simulink model "torqueTest"  (R2020b)
settings: Solver=VariableStepAuto  StartTime=0.0  StopTime=4  FixedStep=0.5  RelTol=1e-3
values from neighbouring files (symbols this model uses):
  X = [x,y,z,Roll,Pitch,Yaw]    [T2RPY.m]
undefined symbols (not defined in the file or in its folder): Y, Z
libraries: sm_lib x75, nesl_utility x25
(part 2 of 2)

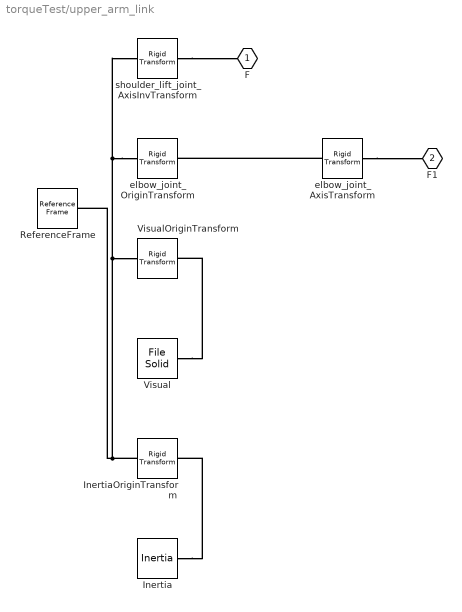
== system torqueTest/upper_arm_link ==
  Inertia : sm_lib/Body Elements/Inertia  InertiaType=Custom  Mass=12.877  MassUnits=kg  CenterOfMass=[0, 0, 0]  CenterOfMassUnits=m  MomentsOfInertia=[0.024695, 0.019038, 0.018496]  MomentsOfInertiaUnits=kg*m^2  ProductsOfInertia=[0.00066134, -6.8716e-08, -8.270400000000001e-09]  ProductsOfInertiaUnits=kg*m^2  GraphicType=None  MarkerShape=Inertia  MarkerSize=20  GraphicVisPropType=SimpleVisualProperties  GraphicDiffuseColor=[0.5 0.5 0.5]  GraphicSpecularColor=[0.5 0.5 0.5 1.0]  GraphicAmbientColor=[0.15 0.15 0.15 1.0]  GraphicEmissiveColor=[0.0 0.0 0.0 1.0]  GraphicShininess=75  GraphicOpacity=1.0
  InertiaOriginTransform : sm_lib/Frames and Transforms/Rigid Transform  TranslationMethod=Cartesian  TranslationStandardOffset=0  TranslationLengthUnit=m  TranslationStandardAxis=+Z  TranslationCartesianOffset=[-5.4357e-07, 0.0032767, 0.12625]  TranslationROffset=0  TranslationROffsetUnits=m  TranslationZOffset=0  TranslationZOffsetUnits=m  TranslationThetaOffset=0  TranslationThetaOffsetUnits=deg  RotationMethod=RotationSequence  RotationAngleUnits=deg  RotationStandardAxis=+Z  RotationAngle=0.0  RotationArbitraryAxis=[0 0 1]  FollAlignAxisA=+X  BaseAlignAxisA=+Y  FollAlignAxisB=+Y  BaseAlignAxisB=+Z  RotationSequenceAxes=BaseAxes  RotationSequence=XYZ  RotationSequenceAngles=[0, 0, 0]  RotationSequenceAnglesUnits=rad  RotationMatrix=[1 0 0; 0 1 0; 0 0 1]
  ReferenceFrame : sm_lib/Frames and Transforms/Reference Frame
  Visual : sm_lib/Body Elements/File Solid  ExtGeomFileName=ROCR6II_URDF_file/meshes/upper_arm_link.STL  UnitType=Custom  ExtGeomFileUnits=m  StepReaderType=HEX  ExportConvexHullGeometry=off  InertiaType=CalculateFromGeometry  Mass=0  MassUnits=kg  CenterOfMass=[0, 0, 0]  CenterOfMassUnits=m  MomentsOfInertia=[0, 0, 0]  MomentsOfInertiaUnits=kg*m^2  ProductsOfInertia=[0, 0, 0]  ProductsOfInertiaUnits=kg*m^2  BasedOnType=Density  Density=1000  DensityUnits=kg/m^3  DoExposeReferenceFrame=on  SerializedFrames=<Frames/>  GraphicType=FromGeometry  MarkerShape=Sphere  MarkerSize=10  GraphicVisPropType=SimpleVisualProperties  GraphicDiffuseColor=[0.7529400000000001, 0.7529400000000001, 0.7529400000000001]  GraphicSpecularColor=[0.5 0.5 0.5 1.0]  GraphicAmbientColor=[0.15 0.15 0.15 1.0]  GraphicEmissiveColor=[0.0 0.0 0.0 1.0]  GraphicShininess=75  GraphicOpacity=1
  VisualOriginTransform : sm_lib/Frames and Transforms/Rigid Transform  TranslationMethod=Cartesian  TranslationStandardOffset=0  TranslationLengthUnit=m  TranslationStandardAxis=+Z  TranslationCartesianOffset=[0, 0, 0]  TranslationROffset=0  TranslationROffsetUnits=m  TranslationZOffset=0  TranslationZOffsetUnits=m  TranslationThetaOffset=0  TranslationThetaOffsetUnits=deg  RotationMethod=RotationSequence  RotationAngleUnits=deg  RotationStandardAxis=+Z  RotationAngle=0.0  RotationArbitraryAxis=[0 0 1]  FollAlignAxisA=+X  BaseAlignAxisA=+Y  FollAlignAxisB=+Y  BaseAlignAxisB=+Z  RotationSequenceAxes=BaseAxes  RotationSequence=XYZ  RotationSequenceAngles=[0, 0, 0]  RotationSequenceAnglesUnits=rad  RotationMatrix=[1 0 0; 0 1 0; 0 0 1]
  elbow_joint_AxisTransform : sm_lib/Frames and Transforms/Rigid Transform  TranslationMethod=Cartesian  TranslationStandardOffset=0  TranslationLengthUnit=m  TranslationStandardAxis=+Z  TranslationCartesianOffset=[0, 0, 0]  TranslationROffset=0  TranslationROffsetUnits=m  TranslationZOffset=0  TranslationZOffsetUnits=m  TranslationThetaOffset=0  TranslationThetaOffsetUnits=deg  RotationMethod=ArbitraryAxis  RotationAngleUnits=rad  RotationStandardAxis=+Z  RotationAngle=1.570796326794897  RotationArbitraryAxis=[-1, 0, 0]  FollAlignAxisA=+X  BaseAlignAxisA=+Y  FollAlignAxisB=+Y  BaseAlignAxisB=+Z  RotationSequenceAxes=FollowerAxes  RotationSequence=XYX  RotationSequenceAngles=[0 0 0]  RotationSequenceAnglesUnits=deg  RotationMatrix=[1 0 0; 0 1 0; 0 0 1]
  elbow_joint_OriginTransform : sm_lib/Frames and Transforms/Rigid Transform  TranslationMethod=Cartesian  TranslationStandardOffset=0  TranslationLengthUnit=m  TranslationStandardAxis=+Z  TranslationCartesianOffset=[0, -0.102, 0.3]  TranslationROffset=0  TranslationROffsetUnits=m  TranslationZOffset=0  TranslationZOffsetUnits=m  TranslationThetaOffset=0  TranslationThetaOffsetUnits=deg  RotationMethod=RotationSequence  RotationAngleUnits=deg  RotationStandardAxis=+Z  RotationAngle=0.0  RotationArbitraryAxis=[0 0 1]  FollAlignAxisA=+X  BaseAlignAxisA=+Y  FollAlignAxisB=+Y  BaseAlignAxisB=+Z  RotationSequenceAxes=BaseAxes  RotationSequence=XYZ  RotationSequenceAngles=[0, 0, 0]  RotationSequenceAnglesUnits=rad  RotationMatrix=[1 0 0; 0 1 0; 0 0 1]
  shoulder_lift_joint_AxisInvTransform : sm_lib/Frames and Transforms/Rigid Transform  TranslationMethod=Cartesian  TranslationStandardOffset=0  TranslationLengthUnit=m  TranslationStandardAxis=+Z  TranslationCartesianOffset=[0, 0, 0]  TranslationROffset=0  TranslationROffsetUnits=m  TranslationZOffset=0  TranslationZOffsetUnits=m  TranslationThetaOffset=0  TranslationThetaOffsetUnits=deg  RotationMethod=ArbitraryAxis  RotationAngleUnits=rad  RotationStandardAxis=+Z  RotationAngle=1.570796326794897  RotationArbitraryAxis=[-1, 0, 0]  FollAlignAxisA=+X  BaseAlignAxisA=+Y  FollAlignAxisB=+Y  BaseAlignAxisB=+Z  RotationSequenceAxes=FollowerAxes  RotationSequence=XYX  RotationSequenceAngles=[0 0 0]  RotationSequenceAnglesUnits=deg  RotationMatrix=[1 0 0; 0 1 0; 0 0 1]
  F : PMIOPort  Side=Left
  F1 : PMIOPort  Port=2  Side=Right
  connections:
  Inertia/RConn1 -- InertiaOriginTransform/RConn1
  elbow_joint_OriginTransform/LConn1 -- shoulder_lift_joint_AxisInvTransform/LConn1 -- InertiaOriginTransform/LConn1 -- ReferenceFrame/RConn1 -- VisualOriginTransform/LConn1
  Visual/RConn1 -- VisualOriginTransform/RConn1
  elbow_joint_AxisTransform/RConn1 -- F1/RConn1
  elbow_joint_AxisTransform/LConn1 -- elbow_joint_OriginTransform/RConn1
  shoulder_lift_joint_AxisInvTransform/RConn1 -- F/RConn1

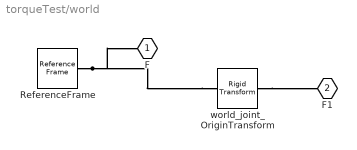
== system torqueTest/world ==
  ReferenceFrame : sm_lib/Frames and Transforms/Reference Frame
  world_joint_OriginTransform : sm_lib/Frames and Transforms/Rigid Transform  TranslationMethod=Cartesian  TranslationStandardOffset=0  TranslationLengthUnit=m  TranslationStandardAxis=+Z  TranslationCartesianOffset=[0, 0, 0]  TranslationROffset=0  TranslationROffsetUnits=m  TranslationZOffset=0  TranslationZOffsetUnits=m  TranslationThetaOffset=0  TranslationThetaOffsetUnits=deg  RotationMethod=RotationSequence  RotationAngleUnits=deg  RotationStandardAxis=+Z  RotationAngle=0.0  RotationArbitraryAxis=[0 0 1]  FollAlignAxisA=+X  BaseAlignAxisA=+Y  FollAlignAxisB=+Y  BaseAlignAxisB=+Z  RotationSequenceAxes=BaseAxes  RotationSequence=XYZ  RotationSequenceAngles=[3.1415926536, 3.1415926536, 0]  RotationSequenceAnglesUnits=rad  RotationMatrix=[1 0 0; 0 1 0; 0 0 1]
  F : PMIOPort  Side=Left
  F1 : PMIOPort  Port=2  Side=Right
  connections:
  world_joint_OriginTransform/LConn1 -- ReferenceFrame/RConn1 -- F/RConn1
  world_joint_OriginTransform/RConn1 -- F1/RConn1

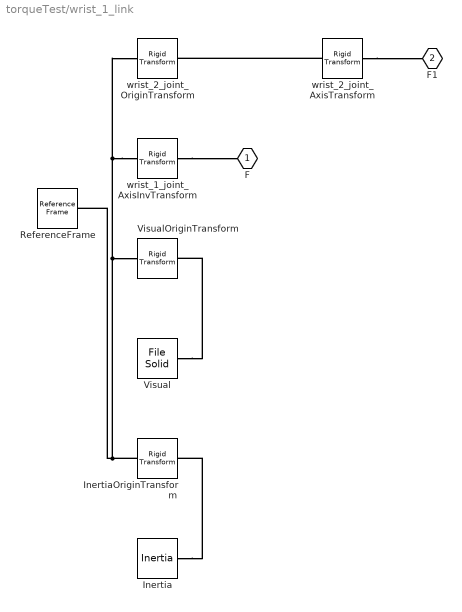
== system torqueTest/wrist_1_link ==
  Inertia : sm_lib/Body Elements/Inertia  InertiaType=Custom  Mass=3.1072  MassUnits=kg  CenterOfMass=[0, 0, 0]  CenterOfMassUnits=m  MomentsOfInertia=[0.0040287, 0.0039406, 0.0018825]  MomentsOfInertiaUnits=kg*m^2  ProductsOfInertia=[9.4145e-05, -2.3481e-09, -7.3158e-09]  ProductsOfInertiaUnits=kg*m^2  GraphicType=None  MarkerShape=Inertia  MarkerSize=20  GraphicVisPropType=SimpleVisualProperties  GraphicDiffuseColor=[0.5 0.5 0.5]  GraphicSpecularColor=[0.5 0.5 0.5 1.0]  GraphicAmbientColor=[0.15 0.15 0.15 1.0]  GraphicEmissiveColor=[0.0 0.0 0.0 1.0]  GraphicShininess=75  GraphicOpacity=1.0
  InertiaOriginTransform : sm_lib/Frames and Transforms/Rigid Transform  TranslationMethod=Cartesian  TranslationStandardOffset=0  TranslationLengthUnit=m  TranslationStandardAxis=+Z  TranslationCartesianOffset=[5.3079e-07, 0.087296, -0.010609]  TranslationROffset=0  TranslationROffsetUnits=m  TranslationZOffset=0  TranslationZOffsetUnits=m  TranslationThetaOffset=0  TranslationThetaOffsetUnits=deg  RotationMethod=RotationSequence  RotationAngleUnits=deg  RotationStandardAxis=+Z  RotationAngle=0.0  RotationArbitraryAxis=[0 0 1]  FollAlignAxisA=+X  BaseAlignAxisA=+Y  FollAlignAxisB=+Y  BaseAlignAxisB=+Z  RotationSequenceAxes=BaseAxes  RotationSequence=XYZ  RotationSequenceAngles=[0, 0, 0]  RotationSequenceAnglesUnits=rad  RotationMatrix=[1 0 0; 0 1 0; 0 0 1]
  ReferenceFrame : sm_lib/Frames and Transforms/Reference Frame
  Visual : sm_lib/Body Elements/File Solid  ExtGeomFileName=ROCR6II_URDF_file/meshes/wrist_1_link.STL  UnitType=Custom  ExtGeomFileUnits=m  StepReaderType=HEX  ExportConvexHullGeometry=off  InertiaType=CalculateFromGeometry  Mass=0  MassUnits=kg  CenterOfMass=[0, 0, 0]  CenterOfMassUnits=m  MomentsOfInertia=[0, 0, 0]  MomentsOfInertiaUnits=kg*m^2  ProductsOfInertia=[0, 0, 0]  ProductsOfInertiaUnits=kg*m^2  BasedOnType=Density  Density=1000  DensityUnits=kg/m^3  DoExposeReferenceFrame=on  SerializedFrames=<Frames/>  GraphicType=FromGeometry  MarkerShape=Sphere  MarkerSize=10  GraphicVisPropType=SimpleVisualProperties  GraphicDiffuseColor=[1, 1, 1]  GraphicSpecularColor=[0.5 0.5 0.5 1.0]  GraphicAmbientColor=[0.15 0.15 0.15 1.0]  GraphicEmissiveColor=[0.0 0.0 0.0 1.0]  GraphicShininess=75  GraphicOpacity=1
  VisualOriginTransform : sm_lib/Frames and Transforms/Rigid Transform  TranslationMethod=Cartesian  TranslationStandardOffset=0  TranslationLengthUnit=m  TranslationStandardAxis=+Z  TranslationCartesianOffset=[0, 0, 0]  TranslationROffset=0  TranslationROffsetUnits=m  TranslationZOffset=0  TranslationZOffsetUnits=m  TranslationThetaOffset=0  TranslationThetaOffsetUnits=deg  RotationMethod=RotationSequence  RotationAngleUnits=deg  RotationStandardAxis=+Z  RotationAngle=0.0  RotationArbitraryAxis=[0 0 1]  FollAlignAxisA=+X  BaseAlignAxisA=+Y  FollAlignAxisB=+Y  BaseAlignAxisB=+Z  RotationSequenceAxes=BaseAxes  RotationSequence=XYZ  RotationSequenceAngles=[0, 0, 0]  RotationSequenceAnglesUnits=rad  RotationMatrix=[1 0 0; 0 1 0; 0 0 1]
  wrist_1_joint_AxisInvTransform : sm_lib/Frames and Transforms/Rigid Transform  TranslationMethod=Cartesian  TranslationStandardOffset=0  TranslationLengthUnit=m  TranslationStandardAxis=+Z  TranslationCartesianOffset=[0, 0, 0]  TranslationROffset=0  TranslationROffsetUnits=m  TranslationZOffset=0  TranslationZOffsetUnits=m  TranslationThetaOffset=0  TranslationThetaOffsetUnits=deg  RotationMethod=ArbitraryAxis  RotationAngleUnits=rad  RotationStandardAxis=+Z  RotationAngle=1.570796326794897  RotationArbitraryAxis=[-1, 0, 0]  FollAlignAxisA=+X  BaseAlignAxisA=+Y  FollAlignAxisB=+Y  BaseAlignAxisB=+Z  RotationSequenceAxes=FollowerAxes  RotationSequence=XYX  RotationSequenceAngles=[0 0 0]  RotationSequenceAnglesUnits=deg  RotationMatrix=[1 0 0; 0 1 0; 0 0 1]
  wrist_2_joint_AxisTransform : sm_lib/Frames and Transforms/Rigid Transform  TranslationMethod=Cartesian  TranslationStandardOffset=0  TranslationLengthUnit=m  TranslationStandardAxis=+Z  TranslationCartesianOffset=[0, 0, 0]  TranslationROffset=0  TranslationROffsetUnits=m  TranslationZOffset=0  TranslationZOffsetUnits=m  TranslationThetaOffset=0  TranslationThetaOffsetUnits=deg  RotationMethod=ArbitraryAxis  RotationAngleUnits=rad  RotationStandardAxis=+Z  RotationAngle=0  RotationArbitraryAxis=[1, 0, 0]  FollAlignAxisA=+X  BaseAlignAxisA=+Y  FollAlignAxisB=+Y  BaseAlignAxisB=+Z  RotationSequenceAxes=FollowerAxes  RotationSequence=XYX  RotationSequenceAngles=[0 0 0]  RotationSequenceAnglesUnits=deg  RotationMatrix=[1 0 0; 0 1 0; 0 0 1]
  wrist_2_joint_OriginTransform : sm_lib/Frames and Transforms/Rigid Transform  TranslationMethod=Cartesian  TranslationStandardOffset=0  TranslationLengthUnit=m  TranslationStandardAxis=+Z  TranslationCartesianOffset=[0, 0.09, 0]  TranslationROffset=0  TranslationROffsetUnits=m  TranslationZOffset=0  TranslationZOffsetUnits=m  TranslationThetaOffset=0  TranslationThetaOffsetUnits=deg  RotationMethod=RotationSequence  RotationAngleUnits=deg  RotationStandardAxis=+Z  RotationAngle=0.0  RotationArbitraryAxis=[0 0 1]  FollAlignAxisA=+X  BaseAlignAxisA=+Y  FollAlignAxisB=+Y  BaseAlignAxisB=+Z  RotationSequenceAxes=BaseAxes  RotationSequence=XYZ  RotationSequenceAngles=[0, 0, 0]  RotationSequenceAnglesUnits=rad  RotationMatrix=[1 0 0; 0 1 0; 0 0 1]
  F : PMIOPort  Side=Left
  F1 : PMIOPort  Port=2  Side=Right
  connections:
  Inertia/RConn1 -- InertiaOriginTransform/RConn1
  wrist_1_joint_AxisInvTransform/LConn1 -- wrist_2_joint_OriginTransform/LConn1 -- InertiaOriginTransform/LConn1 -- ReferenceFrame/RConn1 -- VisualOriginTransform/LConn1
  Visual/RConn1 -- VisualOriginTransform/RConn1
  wrist_1_joint_AxisInvTransform/RConn1 -- F/RConn1
  wrist_2_joint_AxisTransform/RConn1 -- F1/RConn1
  wrist_2_joint_AxisTransform/LConn1 -- wrist_2_joint_OriginTransform/RConn1

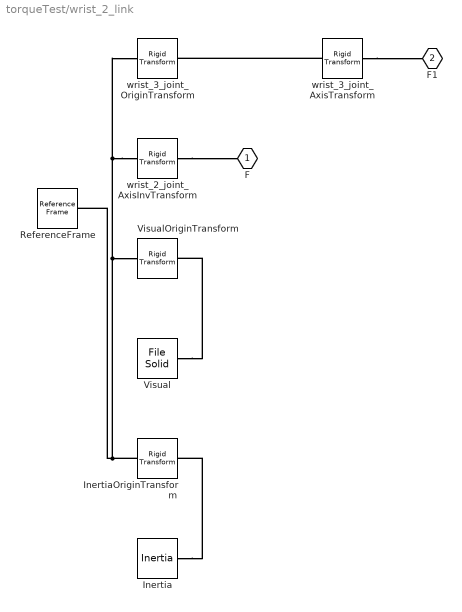
== system torqueTest/wrist_2_link ==
  Inertia : sm_lib/Body Elements/Inertia  InertiaType=Custom  Mass=3.1072  MassUnits=kg  CenterOfMass=[0, 0, 0]  CenterOfMassUnits=m  MomentsOfInertia=[0.0040287, 0.0018825, 0.0039406]  MomentsOfInertiaUnits=kg*m^2  ProductsOfInertia=[9.4145e-05, 7.3e-09, 2.3491e-09]  ProductsOfInertiaUnits=kg*m^2  GraphicType=None  MarkerShape=Inertia  MarkerSize=20  GraphicVisPropType=SimpleVisualProperties  GraphicDiffuseColor=[0.5 0.5 0.5]  GraphicSpecularColor=[0.5 0.5 0.5 1.0]  GraphicAmbientColor=[0.15 0.15 0.15 1.0]  GraphicEmissiveColor=[0.0 0.0 0.0 1.0]  GraphicShininess=75  GraphicOpacity=1.0
  InertiaOriginTransform : sm_lib/Frames and Transforms/Rigid Transform  TranslationMethod=Cartesian  TranslationStandardOffset=0  TranslationLengthUnit=m  TranslationStandardAxis=+Z  TranslationCartesianOffset=[-5.306000000000001e-07, -0.010609, 0.087296]  TranslationROffset=0  TranslationROffsetUnits=m  TranslationZOffset=0  TranslationZOffsetUnits=m  TranslationThetaOffset=0  TranslationThetaOffsetUnits=deg  RotationMethod=RotationSequence  RotationAngleUnits=deg  RotationStandardAxis=+Z  RotationAngle=0.0  RotationArbitraryAxis=[0 0 1]  FollAlignAxisA=+X  BaseAlignAxisA=+Y  FollAlignAxisB=+Y  BaseAlignAxisB=+Z  RotationSequenceAxes=BaseAxes  RotationSequence=XYZ  RotationSequenceAngles=[0, 0, 0]  RotationSequenceAnglesUnits=rad  RotationMatrix=[1 0 0; 0 1 0; 0 0 1]
  ReferenceFrame : sm_lib/Frames and Transforms/Reference Frame
  Visual : sm_lib/Body Elements/File Solid  ExtGeomFileName=ROCR6II_URDF_file/meshes/wrist_2_link.STL  UnitType=Custom  ExtGeomFileUnits=m  StepReaderType=HEX  ExportConvexHullGeometry=off  InertiaType=CalculateFromGeometry  Mass=0  MassUnits=kg  CenterOfMass=[0, 0, 0]  CenterOfMassUnits=m  MomentsOfInertia=[0, 0, 0]  MomentsOfInertiaUnits=kg*m^2  ProductsOfInertia=[0, 0, 0]  ProductsOfInertiaUnits=kg*m^2  BasedOnType=Density  Density=1000  DensityUnits=kg/m^3  DoExposeReferenceFrame=on  SerializedFrames=<Frames/>  GraphicType=FromGeometry  MarkerShape=Sphere  MarkerSize=10  GraphicVisPropType=SimpleVisualProperties  GraphicDiffuseColor=[1, 1, 1]  GraphicSpecularColor=[0.5 0.5 0.5 1.0]  GraphicAmbientColor=[0.15 0.15 0.15 1.0]  GraphicEmissiveColor=[0.0 0.0 0.0 1.0]  GraphicShininess=75  GraphicOpacity=1
  VisualOriginTransform : sm_lib/Frames and Transforms/Rigid Transform  TranslationMethod=Cartesian  TranslationStandardOffset=0  TranslationLengthUnit=m  TranslationStandardAxis=+Z  TranslationCartesianOffset=[0, 0, 0]  TranslationROffset=0  TranslationROffsetUnits=m  TranslationZOffset=0  TranslationZOffsetUnits=m  TranslationThetaOffset=0  TranslationThetaOffsetUnits=deg  RotationMethod=RotationSequence  RotationAngleUnits=deg  RotationStandardAxis=+Z  RotationAngle=0.0  RotationArbitraryAxis=[0 0 1]  FollAlignAxisA=+X  BaseAlignAxisA=+Y  FollAlignAxisB=+Y  BaseAlignAxisB=+Z  RotationSequenceAxes=BaseAxes  RotationSequence=XYZ  RotationSequenceAngles=[0, 0, 0]  RotationSequenceAnglesUnits=rad  RotationMatrix=[1 0 0; 0 1 0; 0 0 1]
  wrist_2_joint_AxisInvTransform : sm_lib/Frames and Transforms/Rigid Transform  TranslationMethod=Cartesian  TranslationStandardOffset=0  TranslationLengthUnit=m  TranslationStandardAxis=+Z  TranslationCartesianOffset=[0, 0, 0]  TranslationROffset=0  TranslationROffsetUnits=m  TranslationZOffset=0  TranslationZOffsetUnits=m  TranslationThetaOffset=0  TranslationThetaOffsetUnits=deg  RotationMethod=ArbitraryAxis  RotationAngleUnits=rad  RotationStandardAxis=+Z  RotationAngle=0  RotationArbitraryAxis=[1, 0, 0]  FollAlignAxisA=+X  BaseAlignAxisA=+Y  FollAlignAxisB=+Y  BaseAlignAxisB=+Z  RotationSequenceAxes=FollowerAxes  RotationSequence=XYX  RotationSequenceAngles=[0 0 0]  RotationSequenceAnglesUnits=deg  RotationMatrix=[1 0 0; 0 1 0; 0 0 1]
  wrist_3_joint_AxisTransform : sm_lib/Frames and Transforms/Rigid Transform  TranslationMethod=Cartesian  TranslationStandardOffset=0  TranslationLengthUnit=m  TranslationStandardAxis=+Z  TranslationCartesianOffset=[0, 0, 0]  TranslationROffset=0  TranslationROffsetUnits=m  TranslationZOffset=0  TranslationZOffsetUnits=m  TranslationThetaOffset=0  TranslationThetaOffsetUnits=deg  RotationMethod=ArbitraryAxis  RotationAngleUnits=rad  RotationStandardAxis=+Z  RotationAngle=1.570796326794897  RotationArbitraryAxis=[-1, 0, 0]  FollAlignAxisA=+X  BaseAlignAxisA=+Y  FollAlignAxisB=+Y  BaseAlignAxisB=+Z  RotationSequenceAxes=FollowerAxes  RotationSequence=XYX  RotationSequenceAngles=[0 0 0]  RotationSequenceAnglesUnits=deg  RotationMatrix=[1 0 0; 0 1 0; 0 0 1]
  wrist_3_joint_OriginTransform : sm_lib/Frames and Transforms/Rigid Transform  TranslationMethod=Cartesian  TranslationStandardOffset=0  TranslationLengthUnit=m  TranslationStandardAxis=+Z  TranslationCartesianOffset=[0, 0, 0.09]  TranslationROffset=0  TranslationROffsetUnits=m  TranslationZOffset=0  TranslationZOffsetUnits=m  TranslationThetaOffset=0  TranslationThetaOffsetUnits=deg  RotationMethod=RotationSequence  RotationAngleUnits=deg  RotationStandardAxis=+Z  RotationAngle=0.0  RotationArbitraryAxis=[0 0 1]  FollAlignAxisA=+X  BaseAlignAxisA=+Y  FollAlignAxisB=+Y  BaseAlignAxisB=+Z  RotationSequenceAxes=BaseAxes  RotationSequence=XYZ  RotationSequenceAngles=[0, 0, 0]  RotationSequenceAnglesUnits=rad  RotationMatrix=[1 0 0; 0 1 0; 0 0 1]
  F : PMIOPort  Side=Left
  F1 : PMIOPort  Port=2  Side=Right
  connections:
  Inertia/RConn1 -- InertiaOriginTransform/RConn1
  wrist_2_joint_AxisInvTransform/LConn1 -- wrist_3_joint_OriginTransform/LConn1 -- InertiaOriginTransform/LConn1 -- ReferenceFrame/RConn1 -- VisualOriginTransform/LConn1
  Visual/RConn1 -- VisualOriginTransform/RConn1
  wrist_2_joint_AxisInvTransform/RConn1 -- F/RConn1
  wrist_3_joint_AxisTransform/RConn1 -- F1/RConn1
  wrist_3_joint_AxisTransform/LConn1 -- wrist_3_joint_OriginTransform/RConn1

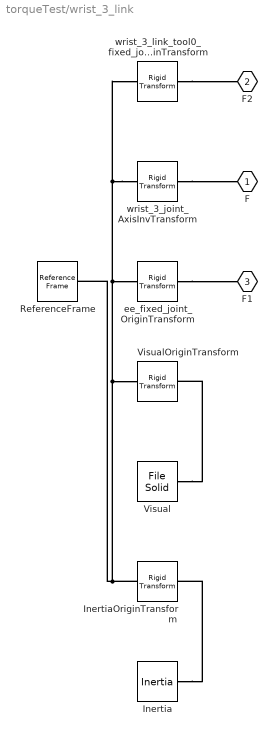
== system torqueTest/wrist_3_link ==
  Inertia : sm_lib/Body Elements/Inertia  InertiaType=Custom  Mass=0.59141  MassUnits=kg  CenterOfMass=[0, 0, 0]  CenterOfMassUnits=m  MomentsOfInertia=[0.0002476, 0.00040058, 0.00024889]  MomentsOfInertiaUnits=kg*m^2  ProductsOfInertia=[4.9238e-06, 1.3425e-10, -2.2015e-14]  ProductsOfInertiaUnits=kg*m^2  GraphicType=None  MarkerShape=Inertia  MarkerSize=20  GraphicVisPropType=SimpleVisualProperties  GraphicDiffuseColor=[0.5 0.5 0.5]  GraphicSpecularColor=[0.5 0.5 0.5 1.0]  GraphicAmbientColor=[0.15 0.15 0.15 1.0]  GraphicEmissiveColor=[0.0 0.0 0.0 1.0]  GraphicShininess=75  GraphicOpacity=1.0
  InertiaOriginTransform : sm_lib/Frames and Transforms/Rigid Transform  TranslationMethod=Cartesian  TranslationStandardOffset=0  TranslationLengthUnit=m  TranslationStandardAxis=+Z  TranslationCartesianOffset=[-1.7174e-09, 0.064961, 2.5473e-05]  TranslationROffset=0  TranslationROffsetUnits=m  TranslationZOffset=0  TranslationZOffsetUnits=m  TranslationThetaOffset=0  TranslationThetaOffsetUnits=deg  RotationMethod=RotationSequence  RotationAngleUnits=deg  RotationStandardAxis=+Z  RotationAngle=0.0  RotationArbitraryAxis=[0 0 1]  FollAlignAxisA=+X  BaseAlignAxisA=+Y  FollAlignAxisB=+Y  BaseAlignAxisB=+Z  RotationSequenceAxes=BaseAxes  RotationSequence=XYZ  RotationSequenceAngles=[0, 0, 0]  RotationSequenceAnglesUnits=rad  RotationMatrix=[1 0 0; 0 1 0; 0 0 1]
  ReferenceFrame : sm_lib/Frames and Transforms/Reference Frame
  Visual : sm_lib/Body Elements/File Solid  ExtGeomFileName=ROCR6II_URDF_file/meshes/wrist_3_link.STL  UnitType=Custom  ExtGeomFileUnits=m  StepReaderType=HEX  ExportConvexHullGeometry=off  InertiaType=CalculateFromGeometry  Mass=0  MassUnits=kg  CenterOfMass=[0, 0, 0]  CenterOfMassUnits=m  MomentsOfInertia=[0, 0, 0]  MomentsOfInertiaUnits=kg*m^2  ProductsOfInertia=[0, 0, 0]  ProductsOfInertiaUnits=kg*m^2  BasedOnType=Density  Density=1000  DensityUnits=kg/m^3  DoExposeReferenceFrame=on  SerializedFrames=<Frames/>  GraphicType=FromGeometry  MarkerShape=Sphere  MarkerSize=10  GraphicVisPropType=SimpleVisualProperties  GraphicDiffuseColor=[0.7529400000000001, 0.7529400000000001, 0.7529400000000001]  GraphicSpecularColor=[0.5 0.5 0.5 1.0]  GraphicAmbientColor=[0.15 0.15 0.15 1.0]  GraphicEmissiveColor=[0.0 0.0 0.0 1.0]  GraphicShininess=75  GraphicOpacity=1
  VisualOriginTransform : sm_lib/Frames and Transforms/Rigid Transform  TranslationMethod=Cartesian  TranslationStandardOffset=0  TranslationLengthUnit=m  TranslationStandardAxis=+Z  TranslationCartesianOffset=[0, 0, 0]  TranslationROffset=0  TranslationROffsetUnits=m  TranslationZOffset=0  TranslationZOffsetUnits=m  TranslationThetaOffset=0  TranslationThetaOffsetUnits=deg  RotationMethod=RotationSequence  RotationAngleUnits=deg  RotationStandardAxis=+Z  RotationAngle=0.0  RotationArbitraryAxis=[0 0 1]  FollAlignAxisA=+X  BaseAlignAxisA=+Y  FollAlignAxisB=+Y  BaseAlignAxisB=+Z  RotationSequenceAxes=BaseAxes  RotationSequence=XYZ  RotationSequenceAngles=[0, 0, 0]  RotationSequenceAnglesUnits=rad  RotationMatrix=[1 0 0; 0 1 0; 0 0 1]
  ee_fixed_joint_OriginTransform : sm_lib/Frames and Transforms/Rigid Transform  TranslationMethod=Cartesian  TranslationStandardOffset=0  TranslationLengthUnit=m  TranslationStandardAxis=+Z  TranslationCartesianOffset=[0, 0.09, 0]  TranslationROffset=0  TranslationROffsetUnits=m  TranslationZOffset=0  TranslationZOffsetUnits=m  TranslationThetaOffset=0  TranslationThetaOffsetUnits=deg  RotationMethod=RotationSequence  RotationAngleUnits=deg  RotationStandardAxis=+Z  RotationAngle=0.0  RotationArbitraryAxis=[0 0 1]  FollAlignAxisA=+X  BaseAlignAxisA=+Y  FollAlignAxisB=+Y  BaseAlignAxisB=+Z  RotationSequenceAxes=BaseAxes  RotationSequence=XYZ  RotationSequenceAngles=[0, 0, 1.57079632679]  RotationSequenceAnglesUnits=rad  RotationMatrix=[1 0 0; 0 1 0; 0 0 1]
  wrist_3_joint_AxisInvTransform : sm_lib/Frames and Transforms/Rigid Transform  TranslationMethod=Cartesian  TranslationStandardOffset=0  TranslationLengthUnit=m  TranslationStandardAxis=+Z  TranslationCartesianOffset=[0, 0, 0]  TranslationROffset=0  TranslationROffsetUnits=m  TranslationZOffset=0  TranslationZOffsetUnits=m  TranslationThetaOffset=0  TranslationThetaOffsetUnits=deg  RotationMethod=ArbitraryAxis  RotationAngleUnits=rad  RotationStandardAxis=+Z  RotationAngle=1.570796326794897  RotationArbitraryAxis=[-1, 0, 0]  FollAlignAxisA=+X  BaseAlignAxisA=+Y  FollAlignAxisB=+Y  BaseAlignAxisB=+Z  RotationSequenceAxes=FollowerAxes  RotationSequence=XYX  RotationSequenceAngles=[0 0 0]  RotationSequenceAnglesUnits=deg  RotationMatrix=[1 0 0; 0 1 0; 0 0 1]
  wrist_3_link_tool0_fixed_joint_OriginTransform : sm_lib/Frames and Transforms/Rigid Transform  TranslationMethod=Cartesian  TranslationStandardOffset=0  TranslationLengthUnit=m  TranslationStandardAxis=+Z  TranslationCartesianOffset=[0, 0.082, 0]  TranslationROffset=0  TranslationROffsetUnits=m  TranslationZOffset=0  TranslationZOffsetUnits=m  TranslationThetaOffset=0  TranslationThetaOffsetUnits=deg  RotationMethod=RotationSequence  RotationAngleUnits=deg  RotationStandardAxis=+Z  RotationAngle=0.0  RotationArbitraryAxis=[0 0 1]  FollAlignAxisA=+X  BaseAlignAxisA=+Y  FollAlignAxisB=+Y  BaseAlignAxisB=+Z  RotationSequenceAxes=BaseAxes  RotationSequence=XYZ  RotationSequenceAngles=[-1.57079632679, 0, 0]  RotationSequenceAnglesUnits=rad  RotationMatrix=[1 0 0; 0 1 0; 0 0 1]
  F : PMIOPort  Side=Left
  F2 : PMIOPort  Port=2  Side=Right
  F1 : PMIOPort  Port=3  Side=Right
  connections:
  Inertia/RConn1 -- InertiaOriginTransform/RConn1
  wrist_3_joint_AxisInvTransform/LConn1 -- wrist_3_link_tool0_fixed_joint_OriginTransform/LConn1 -- InertiaOriginTransform/LConn1 -- ReferenceFrame/RConn1 -- VisualOriginTransform/LConn1 -- ee_fixed_joint_OriginTransform/LConn1
  Visual/RConn1 -- VisualOriginTransform/RConn1
  ee_fixed_joint_OriginTransform/RConn1 -- F1/RConn1
  wrist_3_joint_AxisInvTransform/RConn1 -- F/RConn1
  wrist_3_link_tool0_fixed_joint_OriginTransform/RConn1 -- F2/RConn1

== matlab function torqueTest/Subsystem/trToRPY1 ==
  data: T input; X output
function  X=Tr2Pos(T)
%#codegen
coder.extrinsic('disp'); %Declare disp as extrinsic
    %% 求末端位置
    x=T(1,4);y=T(2,4);z=T(3,4);
    %% 根据X-Y-Z固定角计算
    R=T;rpy=[0,0,0];
    if abs(abs(R(3,1)) - 1) < 0.000001  % when |R31| == 1
    % singularity
        rpy(1) = 0;     % roll is zero
        if R(3,1) < 0
            rpy(3) = -atan2(R(1,2), R(1,3));  % R-Y
        else
            rpy(3) = atan2(-R(1,2), -R(1,3));  % R+Y
        end
        rpy(2) = -asin(R(3,1));
    else
        rpy(1) = atan2(R(3,2), R(3,3));  % R
        rpy(3) = atan2(R(2,1), R(1,1));  % Y

        [~,k] = max(abs( [R(1,1) R(2,1) R(3,2) R(3,3)] ));
        switch k
            case 1
                rpy(2) = -atan(R(3,1)*cos(rpy(3))/R(1,1));
            case 2
                rpy(2) = -atan(R(3,1)*sin(rpy(3))/R(2,1));
            case 3
                rpy(2) = -atan(R(3,1)*sin(rpy(1))/R(3,2));
            case 4
                rpy(2) = -atan(R(3,1)*cos(rpy(1))/R(3,3));
        end
    end
%     RPY=rpy*180/pi;
    RPY=rpy;
    Roll=RPY(1);Pitch=RPY(2);Yaw=RPY(3);
    X=[x,y,z,Roll,Pitch,Yaw];
end

== matlab function torqueTest/Subsystem1/J_0 ==
  data: q input; J output
function J = J(q)
q1=q(1);q2=q(2);q3=q(3);q4=q(4);q5=q(5);q6=q(6);
%J
%    J = J(Q1,Q2,Q3,Q4,Q5)

%    This function was generated by the Symbolic Math Toolbox version 8.6.
%    07-Dec-2021 11:30:25

t2 = cos(q1);
t3 = cos(q2);
t4 = cos(q3);
t5 = cos(q4);
t6 = cos(q5);
t7 = sin(q1);
t8 = sin(q2);
t9 = sin(q3);
t10 = sin(q4);
t11 = sin(q5);
t12 = q2+q3+q4;
t13 = cos(t12);
t14 = sin(t12);
t15 = -t2;
t16 = t6.*(3.9e+1./4.0e+2);
t17 = t5.*(5.7e+1./5.0e+2);
t18 = t10.*(5.7e+1./5.0e+2);
t20 = t5.*t11.*(3.9e+1./4.0e+2);
t21 = t10.*t11.*(3.9e+1./4.0e+2);
t19 = -t18;
t22 = -t20;
t23 = t16+1.065e-1;
t24 = t17+t21;
t25 = t18+t22;
t26 = t4.*t24;
t27 = t9.*t24;
t32 = t19+t20+2.37e+2./1.0e+3;
t28 = t4.*t25;
t29 = t9.*t25;
t30 = -t27;
t33 = t4.*t32;
t34 = t9.*t32;
t31 = -t29;
t35 = t27+t28;
t40 = t26+t34;
t41 = t30+t33;
t44 = -t8.*(t27-t33);
t36 = t26+t31;
t37 = t8.*t35;
t42 = t3.*t40;
t43 = t8.*t40;
t46 = t41+3.3e+1./1.25e+2;
t38 = t3.*t36;
t39 = -t37;
t45 = -t43;
t47 = t3.*t46;
t48 = t8.*t46;
t50 = t42+t44;
t49 = t38+t39;
t51 = t42+t48;
t52 = t45+t47;
J = reshape([t2.*t23-t7.*(t43-t47),t7.*t23+t2.*(t43-t47),0.0,0.0,0.0,1.0,t2.*t51,t7.*t51,t43-t47,t7,t15,0.0,t2.*t50,t7.*t50,t43+t3.*(t27-t33),t7,t15,0.0,-t2.*(t37-t38),-t7.*(t37-t38),t3.*t35+t8.*t36,t7,t15,0.0,t7.*t11.*(-3.9e+1./4.0e+2)-t2.*t6.*t13.*(3.9e+1./4.0e+2),t2.*t11.*(3.9e+1./4.0e+2)-t6.*t7.*t13.*(3.9e+1./4.0e+2),t6.*t14.*(-3.9e+1./4.0e+2),t2.*t14,t7.*t14,-t13,0.0,0.0,0.0,t6.*t7+t11.*t13.*t15,t6.*t15-t7.*t11.*t13,-t11.*t14],[6,6]);


end

== matlab function torqueTest/Subsystem1/J_1 ==
  data: phi input; JaDown3 output; theta input; xi input; J input
function JaDown3 = Jana(phi,theta,xi,J)
om2eulmat=[cos(theta)*cos(xi), -sin(xi), 0;
    cos(theta)*sin(xi),  cos(xi), 0;
    -sin(theta),       0, 1];
omega=J(4:6,:);
JaDown3 = om2eulmat\omega;
end

== matlab function torqueTest/Subsystem1/MATLAB Function ==
  data: JaDown3 input; Jana output; J input
function Jana = fcn(JaDown3,J)
Jana=[J(1:3,:);JaDown3];
end

== matlab function torqueTest/Subsystem1/MATLAB Function1 ==
  data: Jana input; Jadot input; Janadot output; Janaold input
function Janadot = fcn(Jana,Jadot,Janaold)
Jadown3 = Jana - Janaold;
Janadot=[Jadot(1:3,:);Jadown3(4:6,:)];
end

== matlab function torqueTest/Subsystem1/MATLAB Function2 ==
  data: Jana input; Janadot input; dq input; ddX output; ddq input
function ddX = getddX(Jana,Janadot,dq,ddq)
ddX = Janadot * dq + Jana * ddq;

== matlab function torqueTest/Subsystem1/MATLAB Function3 ==
  data: Jana input; dX output; dq input
function dX = getdX(Jana,dq)
dX=Jana*dq;

== matlab function torqueTest/Subsystem1/Pdot1 ==
  data: q input; qdot input; Jadot output
function Jadot = Jadot(q,qdot)
%JADOT
%    JADOT = JADOT(Q1,Q2,Q3,Q4,Q5,Q1DOT,Q2DOT,Q3DOT,Q4DOT,Q5DOT)

%    This function was generated by the Symbolic Math Toolbox version 8.6.
%    07-Dec-2021 14:58:16
q1=q(1);q2=q(2);q3=q(3);q4=q(4);q5=q(5);q6=q(6);
q1dot=qdot(1);q2dot=qdot(2);q3dot=qdot(3);q4dot=qdot(4);q5dot=qdot(5);q6dot=qdot(6);
t2 = cos(q1);
t3 = cos(q2);
t4 = cos(q3);
t5 = cos(q4);
t6 = cos(q5);
t7 = sin(q1);
t8 = sin(q2);
t9 = sin(q3);
t10 = sin(q4);
t11 = sin(q5);
t12 = q2+q3+q4;
t13 = q2dot+q3dot+q4dot;
t14 = cos(t12);
t15 = sin(t12);
t16 = t6.*(3.9e+1./4.0e+2);
t17 = t5.*(5.7e+1./5.0e+2);
t18 = t10.*(5.7e+1./5.0e+2);
t22 = t5.*t11.*(3.9e+1./4.0e+2);
t23 = t10.*t11.*(3.9e+1./4.0e+2);
t24 = q4dot.*t10.*(-5.7e+1./5.0e+2);
t30 = q5dot.*t5.*t6.*(-3.9e+1./4.0e+2);
t19 = -t18;
t20 = q4dot.*t17;
t21 = q4dot.*t18;
t25 = -t22;
t26 = q5dot.*t5.*t16;
t27 = q4dot.*t22;
t28 = q5dot.*t10.*t16;
t29 = q4dot.*t23;
t31 = t16+1.065e-1;
t32 = t17+t23;
t33 = t18+t25;
t34 = t4.*t32;
t35 = t9.*t32;
t46 = t19+t22+2.37e+2./1.0e+3;
t51 = t20+t29+t30;
t52 = t24+t27+t28;
t36 = q3dot.*t34;
t37 = q3dot.*t35;
t38 = t4.*t33;
t39 = t9.*t33;
t42 = -t35;
t47 = t4.*t46;
t48 = t9.*t46;
t53 = t4.*t51;
t54 = t4.*t52;
t55 = t9.*t51;
t56 = t9.*t52;
t40 = q3dot.*t38;
t41 = q3dot.*t39;
t43 = -t37;
t44 = -t39;
t49 = q3dot.*t47;
t50 = q3dot.*t48;
t57 = -t54;
t58 = -t55;
t59 = t35+t38;
t66 = t34+t48;
t67 = t42+t47;
t72 = -t8.*(t35-t47);
t75 = -q2dot.*t3.*(t35-t47);
t45 = -t41;
t60 = t34+t44;
t61 = t8.*t59;
t62 = q2dot.*t3.*t59;
t68 = t3.*t66;
t69 = t8.*t66;
t76 = t67+3.3e+1./1.25e+2;
t85 = t37+t40+t55+t57;
t89 = t36+t50+t53+t56;
t92 = t43+t49+t54+t58;
t94 = -t3.*(t37-t49+t55+t57);
t95 = -t8.*(t37-t49+t55+t57);
t63 = t3.*t60;
t64 = -t61;
t65 = q2dot.*t8.*t60;
t70 = q2dot.*t69;
t71 = q2dot.*t68;
t73 = -t69;
t77 = t3.*t76;
t78 = t8.*t76;
t82 = t68+t72;
t84 = t36+t45+t53+t56;
t87 = t3.*t85;
t90 = t3.*t89;
t91 = t8.*t89;
t74 = -t70;
t79 = q2dot.*t78;
t80 = q2dot.*t77;
t81 = t63+t64;
t83 = t68+t78;
t86 = t73+t77;
t88 = t8.*t84;
t93 = -t91;
t96 = t62+t65+t87+t88;
t97 = t74+t75+t93+t94;
t98 = t71+t79+t90+t95;
t99 = t74+t80+t93+t94;
Jadot = reshape([-t7.*t98-q5dot.*t2.*t11.*(3.9e+1./4.0e+2)-q1dot.*t7.*t31-q1dot.*t2.*(t69-t77),t2.*t98-q5dot.*t7.*t11.*(3.9e+1./4.0e+2)+q1dot.*t2.*t31-q1dot.*t7.*(t69-t77),0.0,-t2.*(t70-t80+t91+t3.*(t37-t49+t55+t57))-q1dot.*t7.*t83,-t7.*(t70-t80+t91+t3.*(t37-t49+t55+t57))+q1dot.*t2.*t83,t98,-t2.*(t70+t91+t3.*(t37-t49+t55+t57)+q2dot.*t3.*(t35-t47))-q1dot.*t7.*t82,-t7.*(t70+t91+t3.*(t37-t49+t55+t57)+q2dot.*t3.*(t35-t47))+q1dot.*t2.*t82,t71+t90+t95+q2dot.*t72,-t2.*t96+q1dot.*t7.*(t61-t63),-t7.*t96-q1dot.*t2.*(t61-t63),q2dot.*t63+q2dot.*t64+t3.*t84-t8.*t85,q1dot.*t2.*t11.*(-3.9e+1./4.0e+2)-q5dot.*t6.*t7.*(3.9e+1./4.0e+2)+q5dot.*t2.*t11.*t14.*(3.9e+1./4.0e+2)+q1dot.*t7.*t14.*t16+t2.*t13.*t15.*t16,q1dot.*t7.*t11.*(-3.9e+1./4.0e+2)+q5dot.*t2.*t16-q1dot.*t2.*t6.*t14.*(3.9e+1./4.0e+2)+q5dot.*t7.*t11.*t14.*(3.9e+1./4.0e+2)+t7.*t13.*t15.*t16,q5dot.*t11.*t15.*(3.9e+1./4.0e+2)-t6.*t13.*t14.*(3.9e+1./4.0e+2),0.0,0.0,0.0],[3,6]);

end

== matlab function torqueTest/Subsystem1/T ==
  data: q input; T output
function T = transion(q)
q1=q(1);q2=q(2);q3=q(3);q4=q(4);q5=q(5);q6=q(6);
t2 = cos(q1);
t3 = cos(q2);
t4 = cos(q3);
t5 = cos(q4);
t6 = cos(q5);
t7 = cos(q6);
t8 = sin(q1);
t9 = sin(q2);
t10 = sin(q3);
t11 = sin(q4);
t12 = sin(q5);
t13 = sin(q6);
t14 = t2.*t3;
t15 = t3.*t4;
t16 = t2.*t6;
t17 = t2.*t9;
t18 = t3.*t8;
t19 = t3.*t10;
t20 = t4.*t9;
t21 = t2.*t12;
t22 = t6.*t8;
t23 = t8.*t9;
t24 = t9.*t10;
t25 = t8.*t12;
t42 = t2.*6.123233995736766e-17;
t43 = t6.*6.123233995736766e-17;
t44 = t8.*6.123233995736766e-17;
t45 = t12.*6.123233995736766e-17;
t26 = -t23;
t27 = -t24;
t28 = -t25;
t29 = t19+t20;
t46 = -t42;
t47 = t14.*6.123233995736766e-17;
t48 = t17.*6.123233995736766e-17;
t49 = t18.*6.123233995736766e-17;
t50 = t23.*6.123233995736766e-17;
t30 = t15+t27;
t31 = t5.*t29;
t32 = t11.*t29;
t51 = -t50;
t52 = t17+t49;
t53 = t18+t48;
t55 = t26+t47;
t33 = t5.*t30;
t34 = t11.*t30;
t35 = -t32;
t54 = t14+t51;
t56 = t10.*t52;
t57 = t10.*t53;
t58 = t4.*t52;
t59 = t4.*t53;
t62 = t10.*t55;
t63 = t4.*t55;
t36 = -t33;
t37 = t31+t34;
t38 = t33+t35;
t60 = t10.*t54;
t61 = t4.*t54;
t65 = -t63;
t70 = t59+t62;
t39 = t6.*t37;
t40 = t12.*t37;
t64 = -t61;
t66 = t6.*(t32+t36).*(-6.123233995736766e-17);
t67 = t12.*(t32+t36).*(-6.123233995736766e-17);
t68 = t58+t60;
t69 = t32+t36+3.749399456654644e-33;
t72 = t57+t65;
t75 = t5.*t70;
t76 = t11.*t70;
t41 = -t40;
t71 = t56+t64;
t73 = t5.*t68;
t74 = t11.*t68;
t79 = t5.*t72;
t80 = t11.*t72;
t83 = t39+t45+t67;
t77 = t5.*t71;
t78 = t11.*t71;
t82 = -t80;
t84 = t41+t43+t66;
t87 = t76+t79;
t81 = -t78;
t85 = t74+t77;
t90 = t75+t82;
t96 = t12.*t87.*6.123233995736766e-17;
t98 = t6.*t87.*6.123233995736766e-17;
t99 = t46+t87;
t86 = t73+t81;
t88 = t6.*t85;
t89 = t12.*t85;
t91 = t6.*t90;
t92 = t12.*t90;
t93 = -t91;
t94 = t44+t86;
t95 = t45.*t86;
t97 = t43.*t86;
t100 = t6.*t86.*(-6.123233995736766e-17);
t103 = t16+t92+t98;
t101 = t22+t89+t100;
t102 = t28+t88+t95;
t104 = t21+t93+t96;
T = reshape([-t13.*t94+t13.*(t22+t89-t97).*6.123233995736766e-17-t7.*(-t25+t88+t12.*t86.*6.123233995736766e-17),t13.*t103.*(-6.123233995736766e-17)-t7.*(t21+t93+t45.*t87)+t13.*(t42-t87),-t13.*t69+t7.*t83-t13.*(t40-t43+t43.*(t32+t36)).*6.123233995736766e-17,0.0,-t7.*t94+t7.*(t22+t89-t97).*6.123233995736766e-17+t13.*(-t25+t88+t12.*t86.*6.123233995736766e-17),t7.*t103.*(-6.123233995736766e-17)+t13.*(t21+t93+t45.*t87)+t7.*(t42-t87),-t7.*t69-t13.*t83-t7.*(t40-t43+t43.*(t32+t36)).*6.123233995736766e-17,0.0,t8.*3.749399456654644e-33+t73.*6.123233995736766e-17-t78.*6.123233995736766e-17+t101,t2.*(-3.749399456654644e-33)-t16+t76.*6.123233995736766e-17+t79.*6.123233995736766e-17-t92-t43.*t87,t32.*6.123233995736766e-17-t33.*6.123233995736766e-17+t84+2.295845021658468e-49,0.0,t8.*1.105e-1-t14.*(3.0./1.0e+1)+t22.*(4.1e+1./5.0e+2)+t23.*1.83697019872103e-17+t56.*(6.9e+1./2.5e+2)-t61.*(6.9e+1./2.5e+2)+t73.*9.000000000000001e-2-t78.*9.000000000000001e-2+t89.*(4.1e+1./5.0e+2)-t6.*t86.*5.021051876504148e-18,t2.*(-1.105e-1)-t16.*(4.1e+1./5.0e+2)-t17.*1.83697019872103e-17-t18.*(3.0./1.0e+1)-t59.*(6.9e+1./2.5e+2)-t62.*(6.9e+1./2.5e+2)+t76.*9.000000000000001e-2+t79.*9.000000000000001e-2-t92.*(4.1e+1./5.0e+2)-t6.*t87.*5.021051876504148e-18,t6.*5.021051876504148e-18-t9.*(3.0./1.0e+1)-t19.*(6.9e+1./2.5e+2)-t20.*(6.9e+1./2.5e+2)+t32.*9.000000000000001e-2-t33.*9.000000000000001e-2-t40.*(4.1e+1./5.0e+2)-t6.*(t32+t36).*5.021051876504148e-18+1.215e-1,1.0],[4,4]);
end

== matlab function torqueTest/Subsystem1/trToRPY1 ==
  data: T input; X output
function  X=Tr2Pos(T)
%#codegen
coder.extrinsic('disp'); %Declare disp as extrinsic
    %% 求末端位置
    x=T(1,4);y=T(2,4);z=T(3,4);
    %% 根据X-Y-Z固定角计算
    R=T;rpy=[0,0,0];
    if abs(abs(R(3,1)) - 1) < 0.000001  % when |R31| == 1
    % singularity
        rpy(1) = 0;     % roll is zero
        if R(3,1) < 0
            rpy(3) = -atan2(R(1,2), R(1,3));  % R-Y
        else
            rpy(3) = atan2(-R(1,2), -R(1,3));  % R+Y
        end
        rpy(2) = -asin(R(3,1));
    else
        rpy(1) = atan2(R(3,2), R(3,3));  % R
        rpy(3) = atan2(R(2,1), R(1,1));  % Y

        [~,k] = max(abs( [R(1,1) R(2,1) R(3,2) R(3,3)] ));
        switch k
            case 1
                rpy(2) = -atan(R(3,1)*cos(rpy(3))/R(1,1));
            case 2
                rpy(2) = -atan(R(3,1)*sin(rpy(3))/R(2,1));
            case 3
                rpy(2) = -atan(R(3,1)*sin(rpy(1))/R(3,2));
            case 4
                rpy(2) = -atan(R(3,1)*cos(rpy(1))/R(3,3));
        end
    end
%     RPY=rpy*180/pi;
    RPY=rpy;
    Roll=RPY(1);Pitch=RPY(2);Yaw=RPY(3);
    X=[x,y,z,Roll,Pitch,Yaw];
end

== matlab function torqueTest/impedent_control1/Admittance Control2 ==
  data: m_M parameter; m_B parameter; m_K parameter; X input; dX input; ddX input; F output double; J_o input
function F = fcn(m_M, m_B, m_K,X,dX,ddX,J_o)

%% control parameter
F = zeros(6,1);
Md = diag(m_M);
Bd = diag(m_B);
Kd = diag(m_K);

F = J_o'*(Md * ddX + Bd * dX + Kd * X');
% F = J_o'*(0 * ddX + 0 * dX + 0 * X');
end

== matlab function torqueTest/J_1 ==
  data: q input; J output
function J = J(q)
q1=q(1);q2=q(2);q3=q(3);q4=q(4);q5=q(5);q6=q(6);
%J
%    J = J(Q1,Q2,Q3,Q4,Q5)

%    This function was generated by the Symbolic Math Toolbox version 8.6.
%    07-Dec-2021 11:30:25

t2 = cos(q1);
t3 = cos(q2);
t4 = cos(q3);
t5 = cos(q4);
t6 = cos(q5);
t7 = sin(q1);
t8 = sin(q2);
t9 = sin(q3);
t10 = sin(q4);
t11 = sin(q5);
t12 = q2+q3+q4;
t13 = cos(t12);
t14 = sin(t12);
t15 = -t2;
t16 = t6.*(3.9e+1./4.0e+2);
t17 = t5.*(5.7e+1./5.0e+2);
t18 = t10.*(5.7e+1./5.0e+2);
t20 = t5.*t11.*(3.9e+1./4.0e+2);
t21 = t10.*t11.*(3.9e+1./4.0e+2);
t19 = -t18;
t22 = -t20;
t23 = t16+1.065e-1;
t24 = t17+t21;
t25 = t18+t22;
t26 = t4.*t24;
t27 = t9.*t24;
t32 = t19+t20+2.37e+2./1.0e+3;
t28 = t4.*t25;
t29 = t9.*t25;
t30 = -t27;
t33 = t4.*t32;
t34 = t9.*t32;
t31 = -t29;
t35 = t27+t28;
t40 = t26+t34;
t41 = t30+t33;
t44 = -t8.*(t27-t33);
t36 = t26+t31;
t37 = t8.*t35;
t42 = t3.*t40;
t43 = t8.*t40;
t46 = t41+3.3e+1./1.25e+2;
t38 = t3.*t36;
t39 = -t37;
t45 = -t43;
t47 = t3.*t46;
t48 = t8.*t46;
t50 = t42+t44;
t49 = t38+t39;
t51 = t42+t48;
t52 = t45+t47;
J = reshape([t2.*t23-t7.*(t43-t47),t7.*t23+t2.*(t43-t47),0.0,0.0,0.0,1.0,t2.*t51,t7.*t51,t43-t47,t7,t15,0.0,t2.*t50,t7.*t50,t43+t3.*(t27-t33),t7,t15,0.0,-t2.*(t37-t38),-t7.*(t37-t38),t3.*t35+t8.*t36,t7,t15,0.0,t7.*t11.*(-3.9e+1./4.0e+2)-t2.*t6.*t13.*(3.9e+1./4.0e+2),t2.*t11.*(3.9e+1./4.0e+2)-t6.*t7.*t13.*(3.9e+1./4.0e+2),t6.*t14.*(-3.9e+1./4.0e+2),t2.*t14,t7.*t14,-t13,0.0,0.0,0.0,t6.*t7+t11.*t13.*t15,t6.*t15-t7.*t11.*t13,-t11.*t14],[6,6]);


end

== matlab function torqueTest/T1 ==
  data: q input; q output
function q = offset(q)
q(2) = q(2) - pi/2;
q(4) = q(4) - pi/2;

end

== matlab function torqueTest/Subsystem/J_0 ==
  data: q input; J output
function J = J(q)
q1=q(1);q2=q(2);q3=q(3);q4=q(4);q5=q(5);q6=q(6);
%J
%    J = J(Q1,Q2,Q3,Q4,Q5)

%    This function was generated by the Symbolic Math Toolbox version 8.6.
%    07-Dec-2021 11:30:25

t2 = cos(q1);
t3 = cos(q2);
t4 = cos(q3);
t5 = cos(q4);
t6 = cos(q5);
t7 = sin(q1);
t8 = sin(q2);
t9 = sin(q3);
t10 = sin(q4);
t11 = sin(q5);
t12 = q2+q3+q4;
t13 = cos(t12);
t14 = sin(t12);
t15 = -t2;
t16 = t6.*(3.9e+1./4.0e+2);
t17 = t5.*(5.7e+1./5.0e+2);
t18 = t10.*(5.7e+1./5.0e+2);
t20 = t5.*t11.*(3.9e+1./4.0e+2);
t21 = t10.*t11.*(3.9e+1./4.0e+2);
t19 = -t18;
t22 = -t20;
t23 = t16+1.065e-1;
t24 = t17+t21;
t25 = t18+t22;
t26 = t4.*t24;
t27 = t9.*t24;
t32 = t19+t20+2.37e+2./1.0e+3;
t28 = t4.*t25;
t29 = t9.*t25;
t30 = -t27;
t33 = t4.*t32;
t34 = t9.*t32;
t31 = -t29;
t35 = t27+t28;
t40 = t26+t34;
t41 = t30+t33;
t44 = -t8.*(t27-t33);
t36 = t26+t31;
t37 = t8.*t35;
t42 = t3.*t40;
t43 = t8.*t40;
t46 = t41+3.3e+1./1.25e+2;
t38 = t3.*t36;
t39 = -t37;
t45 = -t43;
t47 = t3.*t46;
t48 = t8.*t46;
t50 = t42+t44;
t49 = t38+t39;
t51 = t42+t48;
t52 = t45+t47;
J = reshape([t2.*t23-t7.*(t43-t47),t7.*t23+t2.*(t43-t47),0.0,0.0,0.0,1.0,t2.*t51,t7.*t51,t43-t47,t7,t15,0.0,t2.*t50,t7.*t50,t43+t3.*(t27-t33),t7,t15,0.0,-t2.*(t37-t38),-t7.*(t37-t38),t3.*t35+t8.*t36,t7,t15,0.0,t7.*t11.*(-3.9e+1./4.0e+2)-t2.*t6.*t13.*(3.9e+1./4.0e+2),t2.*t11.*(3.9e+1./4.0e+2)-t6.*t7.*t13.*(3.9e+1./4.0e+2),t6.*t14.*(-3.9e+1./4.0e+2),t2.*t14,t7.*t14,-t13,0.0,0.0,0.0,t6.*t7+t11.*t13.*t15,t6.*t15-t7.*t11.*t13,-t11.*t14],[6,6]);


end

== matlab function torqueTest/Subsystem/J_1 ==
  data: phi input; JaDown3 output; theta input; xi input; J input
function JaDown3 = Jana(phi,theta,xi,J)
om2eulmat=[cos(theta)*cos(xi), -sin(xi), 0;
    cos(theta)*sin(xi),  cos(xi), 0;
    -sin(theta),       0, 1];
omega=J(4:6,:);
JaDown3 = om2eulmat\omega;
end

== matlab function torqueTest/Subsystem/MATLAB Function ==
  data: JaDown3 input; Jana output; J input
function Jana = fcn(JaDown3,J)
Jana=[J(1:3,:);JaDown3];
end

== matlab function torqueTest/Subsystem/MATLAB Function1 ==
  data: Jana input; Jadot input; Janadot output; Janaold input
function Janadot = fcn(Jana,Jadot,Janaold)
Jadown3 = Jana - Janaold;
Janadot=[Jadot(1:3,:);Jadown3(4:6,:)];
end

== matlab function torqueTest/Subsystem/MATLAB Function2 ==
  data: Jana input; Janadot input; dq input; ddX output; ddq input
function ddX = getddX(Jana,Janadot,dq,ddq)
ddX = Janadot * dq + Jana * ddq;

== matlab function torqueTest/Subsystem/MATLAB Function3 ==
  data: Jana input; dX output; dq input
function dX = getdX(Jana,dq)
dX=Jana*dq;

== matlab function torqueTest/Subsystem/Pdot1 ==
  data: q input; qdot input; Jadot output
function Jadot = Jadot(q,qdot)
%JADOT
%    JADOT = JADOT(Q1,Q2,Q3,Q4,Q5,Q1DOT,Q2DOT,Q3DOT,Q4DOT,Q5DOT)

%    This function was generated by the Symbolic Math Toolbox version 8.6.
%    07-Dec-2021 14:58:16
q1=q(1);q2=q(2);q3=q(3);q4=q(4);q5=q(5);q6=q(6);
q1dot=qdot(1);q2dot=qdot(2);q3dot=qdot(3);q4dot=qdot(4);q5dot=qdot(5);q6dot=qdot(6);
t2 = cos(q1);
t3 = cos(q2);
t4 = cos(q3);
t5 = cos(q4);
t6 = cos(q5);
t7 = sin(q1);
t8 = sin(q2);
t9 = sin(q3);
t10 = sin(q4);
t11 = sin(q5);
t12 = q2+q3+q4;
t13 = q2dot+q3dot+q4dot;
t14 = cos(t12);
t15 = sin(t12);
t16 = t6.*(3.9e+1./4.0e+2);
t17 = t5.*(5.7e+1./5.0e+2);
t18 = t10.*(5.7e+1./5.0e+2);
t22 = t5.*t11.*(3.9e+1./4.0e+2);
t23 = t10.*t11.*(3.9e+1./4.0e+2);
t24 = q4dot.*t10.*(-5.7e+1./5.0e+2);
t30 = q5dot.*t5.*t6.*(-3.9e+1./4.0e+2);
t19 = -t18;
t20 = q4dot.*t17;
t21 = q4dot.*t18;
t25 = -t22;
t26 = q5dot.*t5.*t16;
t27 = q4dot.*t22;
t28 = q5dot.*t10.*t16;
t29 = q4dot.*t23;
t31 = t16+1.065e-1;
t32 = t17+t23;
t33 = t18+t25;
t34 = t4.*t32;
t35 = t9.*t32;
t46 = t19+t22+2.37e+2./1.0e+3;
t51 = t20+t29+t30;
t52 = t24+t27+t28;
t36 = q3dot.*t34;
t37 = q3dot.*t35;
t38 = t4.*t33;
t39 = t9.*t33;
t42 = -t35;
t47 = t4.*t46;
t48 = t9.*t46;
t53 = t4.*t51;
t54 = t4.*t52;
t55 = t9.*t51;
t56 = t9.*t52;
t40 = q3dot.*t38;
t41 = q3dot.*t39;
t43 = -t37;
t44 = -t39;
t49 = q3dot.*t47;
t50 = q3dot.*t48;
t57 = -t54;
t58 = -t55;
t59 = t35+t38;
t66 = t34+t48;
t67 = t42+t47;
t72 = -t8.*(t35-t47);
t75 = -q2dot.*t3.*(t35-t47);
t45 = -t41;
t60 = t34+t44;
t61 = t8.*t59;
t62 = q2dot.*t3.*t59;
t68 = t3.*t66;
t69 = t8.*t66;
t76 = t67+3.3e+1./1.25e+2;
t85 = t37+t40+t55+t57;
t89 = t36+t50+t53+t56;
t92 = t43+t49+t54+t58;
t94 = -t3.*(t37-t49+t55+t57);
t95 = -t8.*(t37-t49+t55+t57);
t63 = t3.*t60;
t64 = -t61;
t65 = q2dot.*t8.*t60;
t70 = q2dot.*t69;
t71 = q2dot.*t68;
t73 = -t69;
t77 = t3.*t76;
t78 = t8.*t76;
t82 = t68+t72;
t84 = t36+t45+t53+t56;
t87 = t3.*t85;
t90 = t3.*t89;
t91 = t8.*t89;
t74 = -t70;
t79 = q2dot.*t78;
t80 = q2dot.*t77;
t81 = t63+t64;
t83 = t68+t78;
t86 = t73+t77;
t88 = t8.*t84;
t93 = -t91;
t96 = t62+t65+t87+t88;
t97 = t74+t75+t93+t94;
t98 = t71+t79+t90+t95;
t99 = t74+t80+t93+t94;
Jadot = reshape([-t7.*t98-q5dot.*t2.*t11.*(3.9e+1./4.0e+2)-q1dot.*t7.*t31-q1dot.*t2.*(t69-t77),t2.*t98-q5dot.*t7.*t11.*(3.9e+1./4.0e+2)+q1dot.*t2.*t31-q1dot.*t7.*(t69-t77),0.0,-t2.*(t70-t80+t91+t3.*(t37-t49+t55+t57))-q1dot.*t7.*t83,-t7.*(t70-t80+t91+t3.*(t37-t49+t55+t57))+q1dot.*t2.*t83,t98,-t2.*(t70+t91+t3.*(t37-t49+t55+t57)+q2dot.*t3.*(t35-t47))-q1dot.*t7.*t82,-t7.*(t70+t91+t3.*(t37-t49+t55+t57)+q2dot.*t3.*(t35-t47))+q1dot.*t2.*t82,t71+t90+t95+q2dot.*t72,-t2.*t96+q1dot.*t7.*(t61-t63),-t7.*t96-q1dot.*t2.*(t61-t63),q2dot.*t63+q2dot.*t64+t3.*t84-t8.*t85,q1dot.*t2.*t11.*(-3.9e+1./4.0e+2)-q5dot.*t6.*t7.*(3.9e+1./4.0e+2)+q5dot.*t2.*t11.*t14.*(3.9e+1./4.0e+2)+q1dot.*t7.*t14.*t16+t2.*t13.*t15.*t16,q1dot.*t7.*t11.*(-3.9e+1./4.0e+2)+q5dot.*t2.*t16-q1dot.*t2.*t6.*t14.*(3.9e+1./4.0e+2)+q5dot.*t7.*t11.*t14.*(3.9e+1./4.0e+2)+t7.*t13.*t15.*t16,q5dot.*t11.*t15.*(3.9e+1./4.0e+2)-t6.*t13.*t14.*(3.9e+1./4.0e+2),0.0,0.0,0.0],[3,6]);

end

== matlab function torqueTest/Subsystem/T ==
  data: q input; T output
function T = transion(q)
q1=q(1);q2=q(2);q3=q(3);q4=q(4);q5=q(5);q6=q(6);
t2 = cos(q1);
t3 = cos(q2);
t4 = cos(q3);
t5 = cos(q4);
t6 = cos(q5);
t7 = cos(q6);
t8 = sin(q1);
t9 = sin(q2);
t10 = sin(q3);
t11 = sin(q4);
t12 = sin(q5);
t13 = sin(q6);
t14 = t2.*t3;
t15 = t3.*t4;
t16 = t2.*t6;
t17 = t2.*t9;
t18 = t3.*t8;
t19 = t3.*t10;
t20 = t4.*t9;
t21 = t2.*t12;
t22 = t6.*t8;
t23 = t8.*t9;
t24 = t9.*t10;
t25 = t8.*t12;
t42 = t2.*6.123233995736766e-17;
t43 = t6.*6.123233995736766e-17;
t44 = t8.*6.123233995736766e-17;
t45 = t12.*6.123233995736766e-17;
t26 = -t23;
t27 = -t24;
t28 = -t25;
t29 = t19+t20;
t46 = -t42;
t47 = t14.*6.123233995736766e-17;
t48 = t17.*6.123233995736766e-17;
t49 = t18.*6.123233995736766e-17;
t50 = t23.*6.123233995736766e-17;
t30 = t15+t27;
t31 = t5.*t29;
t32 = t11.*t29;
t51 = -t50;
t52 = t17+t49;
t53 = t18+t48;
t55 = t26+t47;
t33 = t5.*t30;
t34 = t11.*t30;
t35 = -t32;
t54 = t14+t51;
t56 = t10.*t52;
t57 = t10.*t53;
t58 = t4.*t52;
t59 = t4.*t53;
t62 = t10.*t55;
t63 = t4.*t55;
t36 = -t33;
t37 = t31+t34;
t38 = t33+t35;
t60 = t10.*t54;
t61 = t4.*t54;
t65 = -t63;
t70 = t59+t62;
t39 = t6.*t37;
t40 = t12.*t37;
t64 = -t61;
t66 = t6.*(t32+t36).*(-6.123233995736766e-17);
t67 = t12.*(t32+t36).*(-6.123233995736766e-17);
t68 = t58+t60;
t69 = t32+t36+3.749399456654644e-33;
t72 = t57+t65;
t75 = t5.*t70;
t76 = t11.*t70;
t41 = -t40;
t71 = t56+t64;
t73 = t5.*t68;
t74 = t11.*t68;
t79 = t5.*t72;
t80 = t11.*t72;
t83 = t39+t45+t67;
t77 = t5.*t71;
t78 = t11.*t71;
t82 = -t80;
t84 = t41+t43+t66;
t87 = t76+t79;
t81 = -t78;
t85 = t74+t77;
t90 = t75+t82;
t96 = t12.*t87.*6.123233995736766e-17;
t98 = t6.*t87.*6.123233995736766e-17;
t99 = t46+t87;
t86 = t73+t81;
t88 = t6.*t85;
t89 = t12.*t85;
t91 = t6.*t90;
t92 = t12.*t90;
t93 = -t91;
t94 = t44+t86;
t95 = t45.*t86;
t97 = t43.*t86;
t100 = t6.*t86.*(-6.123233995736766e-17);
t103 = t16+t92+t98;
t101 = t22+t89+t100;
t102 = t28+t88+t95;
t104 = t21+t93+t96;
T = reshape([-t13.*t94+t13.*(t22+t89-t97).*6.123233995736766e-17-t7.*(-t25+t88+t12.*t86.*6.123233995736766e-17),t13.*t103.*(-6.123233995736766e-17)-t7.*(t21+t93+t45.*t87)+t13.*(t42-t87),-t13.*t69+t7.*t83-t13.*(t40-t43+t43.*(t32+t36)).*6.123233995736766e-17,0.0,-t7.*t94+t7.*(t22+t89-t97).*6.123233995736766e-17+t13.*(-t25+t88+t12.*t86.*6.123233995736766e-17),t7.*t103.*(-6.123233995736766e-17)+t13.*(t21+t93+t45.*t87)+t7.*(t42-t87),-t7.*t69-t13.*t83-t7.*(t40-t43+t43.*(t32+t36)).*6.123233995736766e-17,0.0,t8.*3.749399456654644e-33+t73.*6.123233995736766e-17-t78.*6.123233995736766e-17+t101,t2.*(-3.749399456654644e-33)-t16+t76.*6.123233995736766e-17+t79.*6.123233995736766e-17-t92-t43.*t87,t32.*6.123233995736766e-17-t33.*6.123233995736766e-17+t84+2.295845021658468e-49,0.0,t8.*1.105e-1-t14.*(3.0./1.0e+1)+t22.*(4.1e+1./5.0e+2)+t23.*1.83697019872103e-17+t56.*(6.9e+1./2.5e+2)-t61.*(6.9e+1./2.5e+2)+t73.*9.000000000000001e-2-t78.*9.000000000000001e-2+t89.*(4.1e+1./5.0e+2)-t6.*t86.*5.021051876504148e-18,t2.*(-1.105e-1)-t16.*(4.1e+1./5.0e+2)-t17.*1.83697019872103e-17-t18.*(3.0./1.0e+1)-t59.*(6.9e+1./2.5e+2)-t62.*(6.9e+1./2.5e+2)+t76.*9.000000000000001e-2+t79.*9.000000000000001e-2-t92.*(4.1e+1./5.0e+2)-t6.*t87.*5.021051876504148e-18,t6.*5.021051876504148e-18-t9.*(3.0./1.0e+1)-t19.*(6.9e+1./2.5e+2)-t20.*(6.9e+1./2.5e+2)+t32.*9.000000000000001e-2-t33.*9.000000000000001e-2-t40.*(4.1e+1./5.0e+2)-t6.*(t32+t36).*5.021051876504148e-18+1.215e-1,1.0],[4,4]);
end
